simulink model "power_BuckConverter_led"  (R2021b)
settings: Solver=VariableStepAuto  StartTime=0.0  StopTime=0.7  MaxStep=1e-4  RelTol=1e-4  EnableMultiTasking=on
libraries: spsDiodeLib x13, spsSeriesRLCBranchLib x2, spsCurrentMeasurementLib x1, spsMosfetLib x1, spsPWMGeneratorDCDCLib x1, simulink x1, spsDCVoltageSourceLib x1, spsVoltageMeasurementLib x1, spspowerguiLib x1
settings Model: Creator=The MathWorks, Inc.  LastModifiedBy=caccolillo
settings SolverCC: AlgebraicLoopSolver=TrustRegion  SolverResetMethod=Robust
settings DataIOCC: ReturnWorkspaceOutputs=off
settings OptimizationCC: EfficientFloat2IntCast=on  LifeSpan=inf
settings DebuggingCC: UniqueDataStoreMsg=error  StrictBusMsg=ErrorOnBusTreatedAsVector  SFUnexpectedBacktrackingDiag=warning  SFNoUnconditionalDefaultTransitionDiag=warning  SFExecutionAtInitializationDiag=none  SFMachineParentedDataDiag=warning  ArithmeticOperatorsInVariantConditions=warning
settings SFSimCC: SimUseLocalCustomCode=off  CustomCodeUndefinedFunction=UseInterfaceOnly
settings RTWCC: RTWUseLocalCustomCode=off
settings CodeAppCC: StateflowObjectComments=on
settings GRTTargetCC: TargetLangStandard=C89/C90 (ANSI)
settings ConfigComp: CovMetricSettings=dw  CovSaveCumulativeToWorkspaceVar=on  CovSaveSingleToWorkspaceVar=on  CovExternalEMLEnable=off
settings SimscapeCC: SimscapeNormalizeSystem=off  SimscapeNominalValues={1, 'bar'; 1, 'cm^3/s'; 1, 'bar*kg/s'; 1, 'kJ/kg'; 1, 'kW'; }

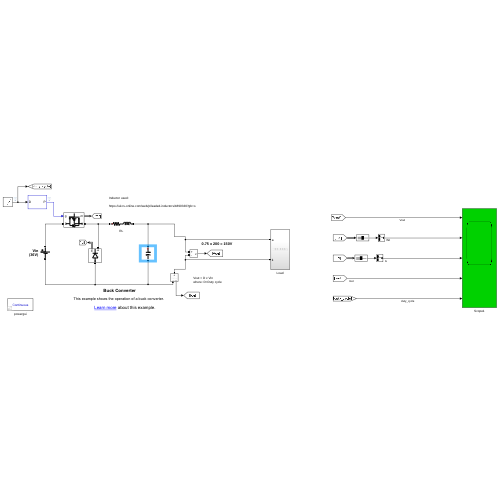
[thumbnail: Simulink's stored preview of the top-level diagram]
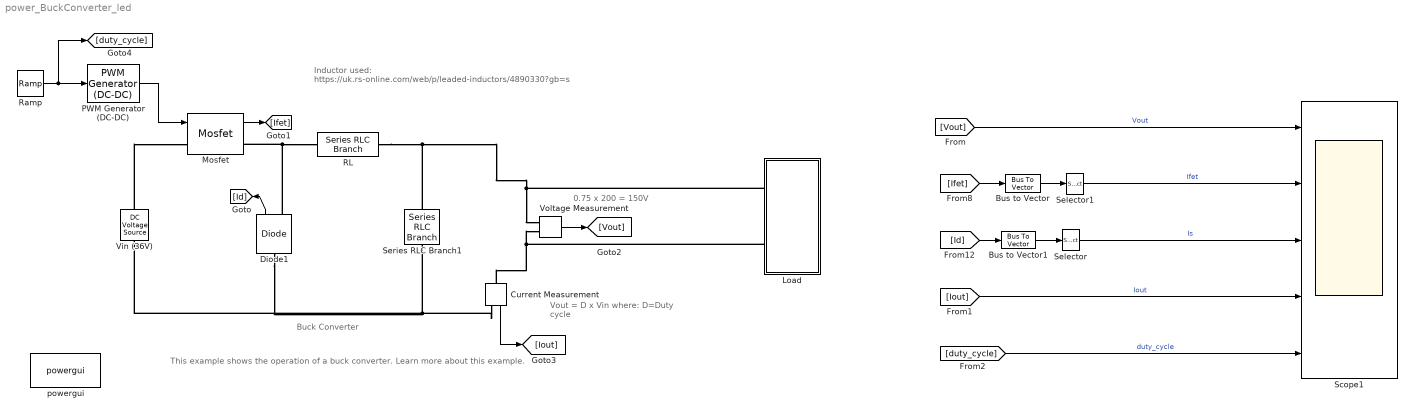
== system power_BuckConverter_led ==
  note: Inductor used:
      |
      | https://uk.rs-online.com/web/p/leaded-inductors/4890330?gb=s
  note: Vout = D x Vin
      | where: D=Duty cycle
  note: 0.75 x 200 = 150V
  note: This example shows the operation of a buck converter.
      |
      | Learn more about this example.
  note: Buck Converter
  Bus to Vector : BusToVector
  Bus to Vector1 : BusToVector
  Current Measurement : spsCurrentMeasurementLib/Current Measurement  PhasorSimulation=off  OutputType=Complex  PSBequivalent=0
  Diode1 : spsDiodeLib/Diode  Ron=1e-3  Lon=0  Vf=0  IC=0  UseSnubber=off  Rs=inf  Cs=inf  Measurements=on
  Load : Subsystem
  Mosfet : spsMosfetLib/Mosfet  Ron=1e-3  Lon=0  Rd=1e-3  Vfd=0  IC=0  Rs=inf  Cs=inf  Measurements=on
  PWM Generator (DC-DC) : spsPWMGeneratorDCDCLib/PWM Generator (DC-DC)  Fsw=150e3  Ts=0
  RL : spsSeriesRLCBranchLib/Series RLC Branch  LConnTagsString=__new0  RConnTagsString=__new0  BranchType=RL  Resistance=0.035  Inductance=68e-3  SetiL0=off  InitialCurrent=0  Capacitance=1e-6  Setx0=off  InitialVoltage=0  Measurements=None
  Ramp : simulink/Sources/Ramp  slope=1  start=0  InitialOutput=0
  Scope1 : Scope  NumInputPorts=5
  Selector : Selector  InputPortWidth=2  IndexOptions=Index vector (dialog)  Indices=1  OutputSizes=1
  Selector1 : Selector  InputPortWidth=2  IndexOptions=Index vector (dialog)  Indices=1  OutputSizes=1
  Series RLC Branch1 : spsSeriesRLCBranchLib/Series RLC Branch  LConnTagsString=__new0  RConnTagsString=__new0  BranchType=C  Resistance=1e-4  Inductance=200e-6  SetiL0=off  InitialCurrent=0  Capacitance=4.7e-6  Setx0=off  InitialVoltage=150  Measurements=None
  Vin (36V) : spsDCVoltageSourceLib/DC Voltage Source  Amplitude=36  Measurements=None
  Voltage Measurement : spsVoltageMeasurementLib/Voltage Measurement  PhasorSimulation=off  OutputType=Complex  PSBequivalent=0
  powergui : spspowerguiLib/powergui  Priority=1  SimulationMode=Continuous  SampleTime=50e-6  frequency=60  Iterations=50  frequencyindice=0  Pbase=100e6  ErrMax=1e-4  UnitsV=kV  UnitsW=MW  buscounter=0  FunctionMessages=off  echomessages=off  EnableUseOfTLC=off  CurrentSourceSwitches=off  DisableSnubberDevices=off  DisableRonSwitches=off  DisableVfSwitches=off  DisplayEquations=off  AutomaticDiscreteSolvers=off  SolverType=Tustin/Backward Euler (TBE)  Interpol=off  ExternalGateDelay=off  methode=off  Ts=100  x0status=blocks  SPID=on  SwTol=0  HookPort=off  NonlinearTolerance=1e-4  nMaxIteration=100  ContinueOnMaxIteration=off  RestoreLinks=warning  ResistiveCurrentMeasurement=off  Frange=[0:2:500]  Ylog=off  Xlog=on  ShowGrid=off  save=off  variable=ZData  structure=0  ZoomFFT=off  StartTime=0.0  cycles=1  DisplayStyle=1  fundamental=60  FreqAxis=off  MaxFrequency=1000  frequencyindicesteady=1  RmsSteady=1  display=off
  wires:
  Diode1/1 -> [Id]
  Voltage Measurement/1 -> [Vout]
  [Ifet] -> Bus to Vector/1
  [Id] -> Bus to Vector1/1
  Mosfet/1 -> [Ifet]
  PWM Generator (DC-DC)/1 -> Mosfet/1
  Selector1/1 -> Scope1/2  "Ifet"
  Selector/1 -> Scope1/3  "Is"
  Ramp/1 -> [duty_cycle], PWM Generator (DC-DC)/1
  [Vout] -> Scope1/1  "Vout"
  Bus to Vector/1 -> Selector1/1
  Bus to Vector1/1 -> Selector/1
  Current Measurement/1 -> [Iout]
  [Iout] -> Scope1/4  "Iout"
  [duty_cycle] -> Scope1/5  "duty_cycle"
  connections:
  Series RLC Branch1/LConn1 -- Load/LConn1 -- Voltage Measurement/LConn1 -- RL/RConn1
  Vin (36V)/RConn1 -- Mosfet/LConn1
  Diode1/RConn1 -- RL/LConn1 -- Mosfet/RConn1
  Diode1/LConn1 -- Vin (36V)/LConn1 -- Current Measurement/RConn1 -- Series RLC Branch1/RConn1
  Current Measurement/LConn1 -- Load/LConn2 -- Voltage Measurement/LConn2

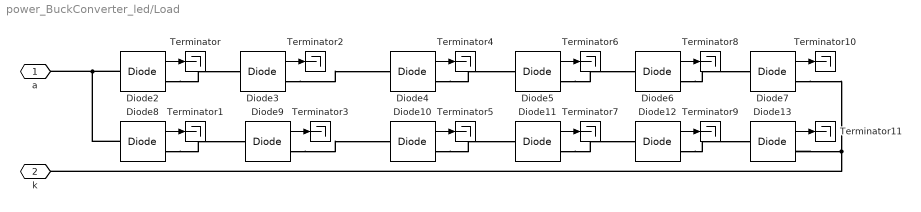
== system power_BuckConverter_led/Load ==
  Diode{2..13} (12 alike) : spsDiodeLib/Diode  Ron=1e-3  Lon=0  Vf=3.3  IC=0  UseSnubber=off  Rs=inf  Cs=inf  Measurements=on
  Terminator{,1..11} (12 alike) : Terminator
  a : PMIOPort  Side=Left
  k : PMIOPort  Port=2  Side=Left
  wires:
  Diode11/1 -> Terminator7/1
  Diode13/1 -> Terminator11/1
  Diode2/1 -> Terminator/1
  Diode7/1 -> Terminator10/1
  Diode3/1 -> Terminator2/1
  Diode6/1 -> Terminator8/1
  Diode12/1 -> Terminator9/1
  Diode8/1 -> Terminator1/1
  Diode5/1 -> Terminator6/1
  Diode10/1 -> Terminator5/1
  Diode9/1 -> Terminator3/1
  Diode4/1 -> Terminator4/1
  connections:
  Diode4/RConn1 -- Diode5/LConn1
  Diode9/RConn1 -- Diode10/LConn1
  Diode8/RConn1 -- Diode9/LConn1
  Diode3/RConn1 -- Diode4/LConn1
  Diode6/RConn1 -- Diode7/LConn1
  Diode2/RConn1 -- Diode3/LConn1
  Diode8/LConn1 -- a/RConn1 -- Diode2/LConn1
  Diode11/RConn1 -- Diode12/LConn1
  Diode10/RConn1 -- Diode11/LConn1
  Diode13/RConn1 -- Diode7/RConn1 -- k/RConn1
  Diode5/RConn1 -- Diode6/LConn1
  Diode12/RConn1 -- Diode13/LConn1
